simulink model "lookupTableDynamic_TestGen28"  (R2017b)
settings: Solver=FixedStepDiscrete  StartTime=0.0  StopTime=10.0  RelTol=1e-3
libraries: simulink x1
settings Model: Creator=ktrinh  LastModifiedBy=ktrinh
settings DebuggingCC: ParameterOverflowMsg=none

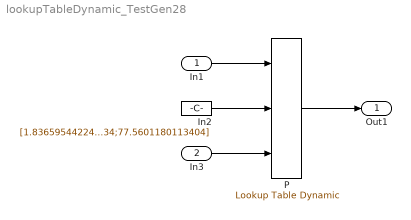
== system lookupTableDynamic_TestGen28 ==
  In1 : Inport  OutMin=0  OutMax=80  OutDataTypeStr=uint8  PortDimensions=1
  In3 : Inport  Port=2  PortDimensions=5
  In2 : Constant  Value=[1.83659544224091;4.48831146652996;53.5194177485047;74.3412914691534;77.5601180113404]  OutDataTypeStr=uint8
  P : simulink/Lookup Tables/Lookup Table Dynamic  LookUpMeth=Use Input Below  OutDataType=fixdt('double')  OutScaling=[]  OutputDataTypeScalingMode=Specify via dialog  OutDataTypeStr=double  RndMeth=Ceiling  DoSatur=off
      settings: SourceProductName=Simulink
  Out1 : Outport
  wires:
  In1/1 -> P/1
  In2/1 -> P/2
  In3/1 -> P/3
  P/1 -> Out1/1
